simulink model "STOP"  (R2018b)
settings: Solver=FixedStepAuto  StartTime=0.0  StopTime=inf  RelTol=1e-3  EnableMultiTasking=on
undefined symbols (not defined in the file or in its folder): Green, led0
libraries: raspberrypilib x5, hdlsllib x2, simulink x1, embdlinuxlib x1
settings Model: SimulationMode=external  Creator=Iansweeney  LastModifiedBy=Iansweeney
settings SolverCC: PositivePriorityOrder=on
settings OptimizationCC: EnhancedBackFolding=on  PassReuseOutputArgsAs=Individual arguments  MaxStackSize=64  OptimizeBlockOrder=speed  DifferentSizesBufferReuse=on  OptimizationCustomize=off
settings DebuggingCC: ParameterTunabilityLossMsg=error
settings HardwareCC: ProdBitPerPointer=32  ProdBitPerSizeT=32  ProdBitPerPtrDiffT=32  ProdLargestAtomicInteger=Long  ProdLargestAtomicFloat=Double  ProdWordSize=32  ProdHWDeviceType=ARM Compatible->ARM Cortex  UseEmbeddedCoderFeatures=off  UseSimulinkCoderFeatures=off
settings SFSimCC: MATLABDynamicMemAlloc=off
settings RTWCC: SystemTargetFile=ert.tlc  HardwareBoard=Raspberry Pi  TLCOptions="-aInlineSetEventsForThisBaseRateFcn=TLC_FALSE -aSuppressMultiTaskScheduler=TLC_FALSE  -aRateBasedStepFcn=0"  TemplateMakefile=ert_default_tmf  GenerateReport=on  Toolchain=GNU GCC Raspberry Pi  BuildConfiguration=Faster Runs  IncludeHyperlinkInReport=on  LaunchReport=on  GenerateTraceInfo=on  GenerateTraceReport=on  GenerateTraceReportSl=on  GenerateTraceReportSf=on  GenerateTraceReportEml=on
settings CodeAppCC: ForceParamTrailComments=on  IgnoreCustomStorageClasses=off  OperatorAnnotations=on  SimulinkDataObjDesc=on  SFDataObjDesc=on  MangleLength=10  InsertBlockDesc=on
settings ERTTargetCC: SupportNonInlinedSFcns=on  SupportVariableSizeSignals=on

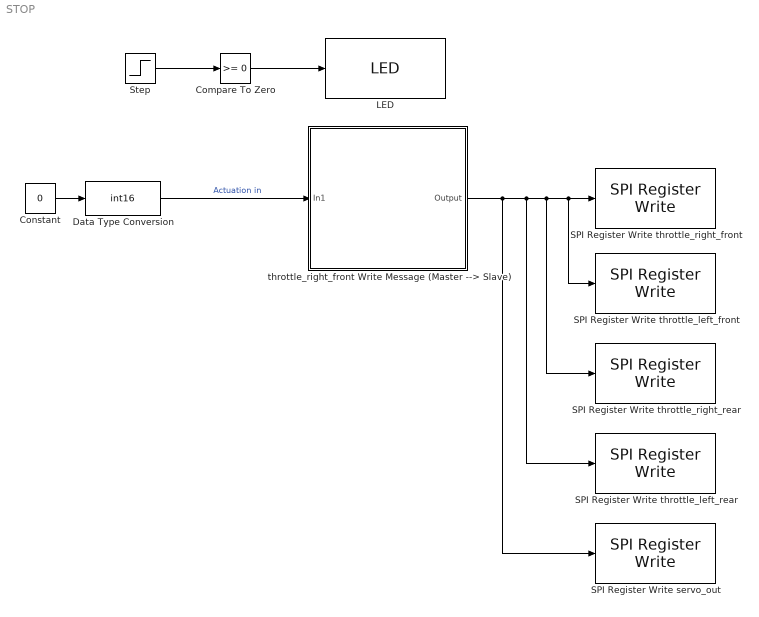
== system STOP ==
  Compare To Zero : simulink/Logic and Bit Operations/Compare To Zero  relop=>=  OutDataTypeStr=boolean
  Constant : Constant  Value=0
  Data Type Conversion : DataTypeConversion  OutDataTypeStr=int16  RndMeth=Nearest  LockScale=on
  LED : embdlinuxlib/LED  board=Pi 3 Model B  led=led0 (Green)  blockPlatform=Raspberry Pi
      settings: SourceProductName=Simulink Support Package for Raspberry Pi Hardware  SourceProductBaseCode=RASPPI
  "SPI Register Write servo_out " : raspberrypilib/SPI Register Write  BoardProperty=Pi 3 Model B  SPIModule=uint32(0)  Mode=Master  BusSpeed=1000000  Pin=SPI0_CE1  FirstBitToTransfer=Most significant bit (MSB)  ClockMode=0  BlockFunction=Write  RegisterAddress=38  OutputDataType=int8  OutputDataLength=1
      settings: SourceProductName=Simulink Support Package for Raspberry Pi Hardware  SourceProductBaseCode=RASPPI
  SPI Register Write throttle_left_front : raspberrypilib/SPI Register Write  BoardProperty=Pi 3 Model B  SPIModule=uint32(0)  Mode=Master  BusSpeed=1000000  Pin=SPI0_CE1  FirstBitToTransfer=Most significant bit (MSB)  ClockMode=0  BlockFunction=Write  RegisterAddress=32  OutputDataType=int8  OutputDataLength=1
      settings: SourceProductName=Simulink Support Package for Raspberry Pi Hardware  SourceProductBaseCode=RASPPI
  SPI Register Write throttle_left_rear : raspberrypilib/SPI Register Write  BoardProperty=Pi 3 Model B  SPIModule=uint32(0)  Mode=Master  BusSpeed=1000000  Pin=SPI0_CE1  FirstBitToTransfer=Most significant bit (MSB)  ClockMode=0  BlockFunction=Write  RegisterAddress=36  OutputDataType=int8  OutputDataLength=1
      settings: SourceProductName=Simulink Support Package for Raspberry Pi Hardware  SourceProductBaseCode=RASPPI
  SPI Register Write throttle_right_front : raspberrypilib/SPI Register Write  BoardProperty=Pi 3 Model B  SPIModule=uint32(0)  Mode=Master  BusSpeed=1000000  Pin=SPI0_CE1  FirstBitToTransfer=Most significant bit (MSB)  ClockMode=0  BlockFunction=Write  RegisterAddress=30  OutputDataType=int8  OutputDataLength=1
      settings: SourceProductName=Simulink Support Package for Raspberry Pi Hardware  SourceProductBaseCode=RASPPI
  SPI Register Write throttle_right_rear : raspberrypilib/SPI Register Write  BoardProperty=Pi 3 Model B  SPIModule=uint32(0)  Mode=Master  BusSpeed=1000000  Pin=SPI0_CE1  FirstBitToTransfer=Most significant bit (MSB)  ClockMode=0  BlockFunction=Write  RegisterAddress=34  OutputDataType=int8  OutputDataLength=1
      settings: SourceProductName=Simulink Support Package for Raspberry Pi Hardware  SourceProductBaseCode=RASPPI
  Step : Step  SampleTime=0
  throttle_right_front Write Message (Master --> Slave) : Subsystem
  wires:
  Compare To Zero/1 -> LED/1
  Step/1 -> Compare To Zero/1
  Data Type Conversion/1 -> throttle_right_front Write Message (Master --> Slave)/1(In1)  "Actuation in"
  throttle_right_front Write Message (Master --> Slave)/1(Output) -> "SPI Register Write servo_out "/1, SPI Register Write throttle_left_rear/1, SPI Register Write throttle_right_rear/1, SPI Register Write throttle_left_front/1, SPI Register Write throttle_right_front/1
  Constant/1 -> Data Type Conversion/1

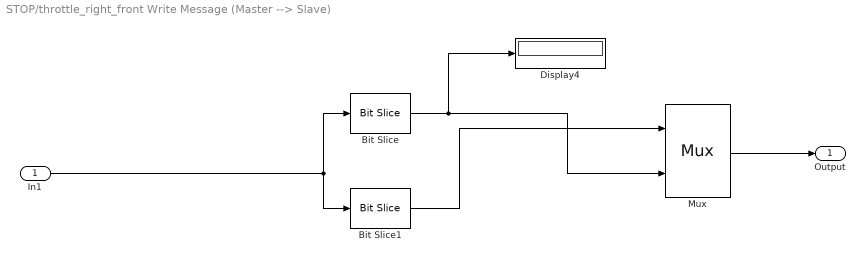
== system STOP/throttle_right_front Write Message (Master --> Slave) ==
  In1 : Inport
  Bit Slice : hdlsllib/Logic and Bit Operations/Bit Slice  lidx=15  ridx=8
  Bit Slice1 : hdlsllib/Logic and Bit Operations/Bit Slice  lidx=7  ridx=0
  Display4 : Display
  Mux : Mux  Inputs=2
      settings: DisplayOption=signals
  Output : Outport
  wires:
  Mux/1 -> Output/1
  Bit Slice/1 -> Display4/1, Mux/2
  Bit Slice1/1 -> Mux/1
  In1/1 -> Bit Slice/1, Bit Slice1/1
